simulink model "GCI_Ctrl_PLL_C2000"  (R2024a)
settings: Solver=FixedStepDiscrete  StartTime=0.0  StopTime=8  FixedStep=Sim.ContSampleTime  RelTol=1e-3  EnableMultiTasking=on
values from neighbouring files (symbols this model uses):
  ADPTV = 1.3912    [ModelDD.sldd]
  Ctrl = 0    [ModelDD.sldd]
  EnableMonitors = 0    [ModelDD.sldd]
  FrcPwr = 1    [ModelDD.sldd]
  IdSp = 0.0    [ModelDD.sldd]
  IqSp = 0.0    [ModelDD.sldd]
  ModReq = 1    [ModelDD.sldd]
  PorISel = 0    [ModelDD.sldd]
  PSp = 0.0    [ModelDD.sldd]
  QSp = 0.0    [ModelDD.sldd]
  Sim : value not decoded    [ModelDD.sldd]
  Test = 0    [ModelDD.sldd]
  Var = 650.0    [ModelDD.sldd]
undefined symbols (not defined in the file or in its folder): DiscIntNeverNeededParam, Down, GPTRIP1SEL, GPTRIP2SEL, magnitude, P, TZ1, TZ2, Up
libraries: simulink x38, c2837xDlib x22, c2802xlib x15, slpidlib x9, spsMeanLib x9, spsCurrentMeasurementLib x7, spsThreePhaseVIMeasurementLib x5, spsVoltageMeasurementLib x5, spsTHDLib x4, spsSeriesRLCBranchLib x4, svdutilitieslib x3, c280xlib x3
(part 4 of 11)

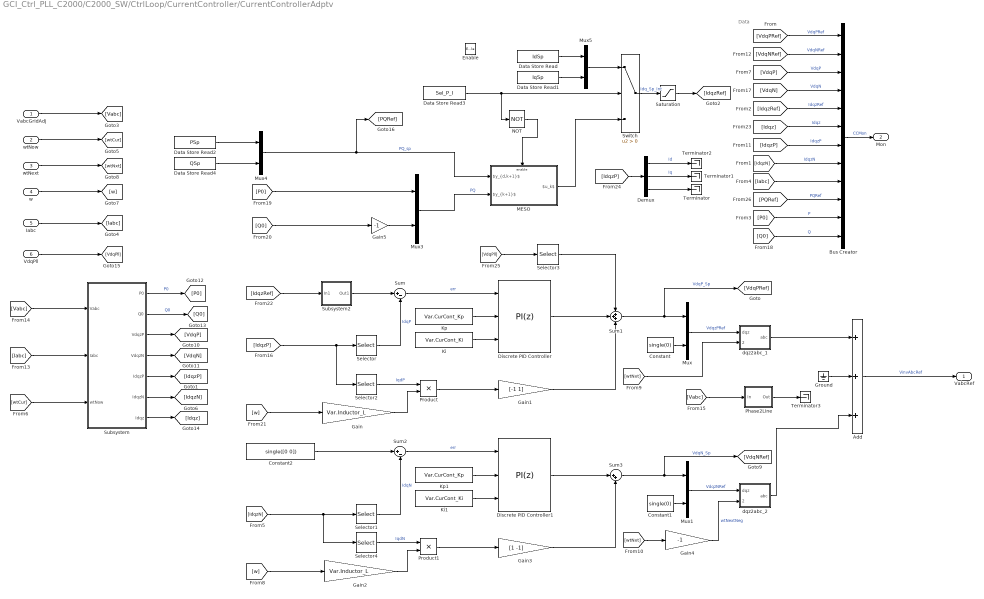
== system GCI_Ctrl_PLL_C2000/C2000_SW/CtrlLoop/CurrentController/CurrentControllerAdptv ==
  note: Data
  VabcGridAdj : Inport
  wtNow : Inport  Port=2
  wtNext : Inport  Port=3
  w : Inport  Port=4
  Iabc : Inport  Port=5
  VdqPll : Inport  Port=6
  Enable : EnablePort  StatesWhenEnabling=reset
  Add : Sum  Inputs=+++
  Bus Creator : BusCreator  Inputs=12
  Constant : Constant  Value=single(0)
  Constant1 : Constant  Value=single(0)
  Constant2 : Constant  Value=single([0 0])
  Data Store Read : DataStoreRead  DataStoreName=IdSp  IndexOptions=Index vector (dialog)  Indices=1  OutputSizes=1
  Data Store Read1 : DataStoreRead  DataStoreName=IqSp  IndexOptions=Index vector (dialog)  Indices=1  OutputSizes=1
  Data Store Read2 : DataStoreRead  DataStoreName=PSp  IndexOptions=Index vector (dialog)  Indices=1  OutputSizes=1
  Data Store Read3 : DataStoreRead  DataStoreName=Sel_P_I  IndexOptions=Index vector (dialog)  Indices=1  OutputSizes=1
  Data Store Read4 : DataStoreRead  DataStoreName=QSp  IndexOptions=Index vector (dialog)  Indices=1  OutputSizes=1
  Demux : Demux  Outputs=3
  Discrete PID Controller : slpidlib/PID Controller  Controller=PI  Form=Parallel  TimeDomain=Discrete-time  UseExternalTs=off  SampleTime=-1  IntegratorMethod=Forward Euler  FilterMethod=Forward Euler  ControllerParametersSource=external  P=1  I=1  UseKiTs=off  D=0  UseExternalDerivativeSource=off  N=100  UseFilter=on  TunerSelectOption=Transfer Function Based (PID Tuner App)  InitialConditionSource=internal  InitialConditionForIntegrator=0  InitialConditionForFilter=0  DifferentiatorICPrevScaledInput=0  ExternalReset=none  TrackingMode=off  Kt=1  LimitOutput=on  SatLimitsSource=internal  UpperSaturationLimit=Var.CurCont_MaxVdVq  LowerSaturationLimit=-Var.CurCont_MaxVdVq  LinearizeAsGain=on  AntiWindupMode=clamping  Kb=1  LimitIntegrator=off  UpperIntegratorSaturationLimit=inf  LowerIntegratorSaturationLimit=-inf  POutMin=[]  POutMax=[]  IOutMin=[]  IOutMax=[]  DOutMin=[]  DOutMax=[]  NOutMin=[]  NOutMax=[]  SumOutMin=[]  SumOutMax=[]  SaturationOutMin=[]  SaturationOutMax=[]  PParamMin=[]  PParamMax=[]  IParamMin=[]  IParamMax=[]  DParamMin=[]  DParamMax=[]  NParamMin=[]  NParamMax=[]  KbParamMin=[]  KbParamMax=[]  KtParamMin=[]  KtParamMax=[]  KbOutMin=[]  KbOutMax=[]  KtOutMin=[]  KtOutMax=[]  IntegratorOutMin=[]  IntegratorOutMax=[]  FilterOutMin=[]  FilterOutMax=[]  SumI1OutMin=[]  SumI1OutMax=[]  SumI2OutMin=[]  SumI2OutMax=[]  SumI3OutMin=[]  SumI3OutMax=[]  SumI4OutMin=[]  SumI4OutMax=[]  SumDOutMin=[]  SumDOutMax=[]  DifferentiatorOutMin=[]  DifferentiatorOutMax=[]  FilterDiffOutCoefMin=[]  FilterDiffOutCoefMax=[]  ReciprocalOutMin=[]  ReciprocalOutMax=[]  SumDenOutMin=[]  SumDenOutMax=[]  SumNumOutMin=[]  SumNumOutMax=[]  DivideOutMin=[]  DivideOutMax=[]  UdiffTsProdOutMin=[]  UdiffTsProdOutMax=[]  NTsProdOutMin=[]  NTsProdOutMax=[]  UintegralTsProdOutMin=[]  UintegralTsProdOutMax=[]  UngainTsProdOutMin=[]  UngainTsProdOutMax=[]  ClampingZeroOutDataTypeStr=Inherit: Inherit via back propagation  ClampingZeroOutMin=[]  ClampingZeroOutMax=[]  FilterDenConstantOutDataTypeStr=Inherit: Inherit via back propagation  FilterDenConstantOutMin=[]  FilterDenConstantOutMax=[]  PCopyOutDataTypeStr=Inherit: Inherit via back propagation  PCopyOutMin=[]  PCopyOutMax=[]  NCopyOutDataTypeStr=Inherit: Inherit via back propagation  NCopyOutMin=[]  NCopyOutMax=[]  IntegratorContinuousStateAttributes=''  IntegratorStateMustResolveToSignalObject=off  IntegratorRTWStateStorageClass=Auto  FilterContinuousStateAttributes=''  FilterStateMustResolveToSignalObject=off  FilterRTWStateStorageClass=Auto  ParallelPVariant=ExternalParameters  IdealPVariant=Disabled  IVariant=ExternalParameters  DVariant=Disabled  IntegratorVariant=Discrete  SatVariant=Enabled  AWVariant=DiscClampingParallel  PCopyVariant=Disabled  TRVariant=Disabled  FdbkBlocksVariant=Forward  IdealPFdbkVariant=Disabled  SatFdbkVariant=Disabled  DerivativeFilterVariant=Disabled  NVariant=Disabled  NCopyVariant=Disabled_SignalSpec  FilterICVariant=Disabled  IntegratorICVariant=InternalICs  ExternalResetVariant=Disabled  TRSumVariant=Passthrough  SumFdbkVariant=Disabled  SumVariant=Sum_PI  TsampFilterVariant=InternalTs  TsampNgainVariant=Passthrough  TsampIntegralVariant=Disabled_SignalSpec  ExternalSaturationOutDataTypeStr=Inherit: Same as second input  DerivativeSourceVariant=Disabled
  Discrete PID Controller1 : slpidlib/PID Controller  Controller=PI  Form=Parallel  TimeDomain=Discrete-time  UseExternalTs=off  SampleTime=-1  IntegratorMethod=Forward Euler  FilterMethod=Forward Euler  ControllerParametersSource=external  P=1  I=1  UseKiTs=off  D=0  UseExternalDerivativeSource=off  N=100  UseFilter=on  TunerSelectOption=Transfer Function Based (PID Tuner App)  InitialConditionSource=internal  InitialConditionForIntegrator=0  InitialConditionForFilter=0  DifferentiatorICPrevScaledInput=0  ExternalReset=none  TrackingMode=off  Kt=1  LimitOutput=on  SatLimitsSource=internal  UpperSaturationLimit=Var.CurCont_MaxVdVq  LowerSaturationLimit=-Var.CurCont_MaxVdVq  LinearizeAsGain=on  AntiWindupMode=clamping  Kb=1  LimitIntegrator=off  UpperIntegratorSaturationLimit=inf  LowerIntegratorSaturationLimit=-inf  POutMin=[]  POutMax=[]  IOutMin=[]  IOutMax=[]  DOutMin=[]  DOutMax=[]  NOutMin=[]  NOutMax=[]  SumOutMin=[]  SumOutMax=[]  SaturationOutMin=[]  SaturationOutMax=[]  PParamMin=[]  PParamMax=[]  IParamMin=[]  IParamMax=[]  DParamMin=[]  DParamMax=[]  NParamMin=[]  NParamMax=[]  KbParamMin=[]  KbParamMax=[]  KtParamMin=[]  KtParamMax=[]  KbOutMin=[]  KbOutMax=[]  KtOutMin=[]  KtOutMax=[]  IntegratorOutMin=[]  IntegratorOutMax=[]  FilterOutMin=[]  FilterOutMax=[]  SumI1OutMin=[]  SumI1OutMax=[]  SumI2OutMin=[]  SumI2OutMax=[]  SumI3OutMin=[]  SumI3OutMax=[]  SumI4OutMin=[]  SumI4OutMax=[]  SumDOutMin=[]  SumDOutMax=[]  DifferentiatorOutMin=[]  DifferentiatorOutMax=[]  FilterDiffOutCoefMin=[]  FilterDiffOutCoefMax=[]  ReciprocalOutMin=[]  ReciprocalOutMax=[]  SumDenOutMin=[]  SumDenOutMax=[]  SumNumOutMin=[]  SumNumOutMax=[]  DivideOutMin=[]  DivideOutMax=[]  UdiffTsProdOutMin=[]  UdiffTsProdOutMax=[]  NTsProdOutMin=[]  NTsProdOutMax=[]  UintegralTsProdOutMin=[]  UintegralTsProdOutMax=[]  UngainTsProdOutMin=[]  UngainTsProdOutMax=[]  ClampingZeroOutDataTypeStr=Inherit: Inherit via back propagation  ClampingZeroOutMin=[]  ClampingZeroOutMax=[]  FilterDenConstantOutDataTypeStr=Inherit: Inherit via back propagation  FilterDenConstantOutMin=[]  FilterDenConstantOutMax=[]  PCopyOutDataTypeStr=Inherit: Inherit via back propagation  PCopyOutMin=[]  PCopyOutMax=[]  NCopyOutDataTypeStr=Inherit: Inherit via back propagation  NCopyOutMin=[]  NCopyOutMax=[]  IntegratorContinuousStateAttributes=''  IntegratorStateMustResolveToSignalObject=off  IntegratorRTWStateStorageClass=Auto  FilterContinuousStateAttributes=''  FilterStateMustResolveToSignalObject=off  FilterRTWStateStorageClass=Auto  ParallelPVariant=ExternalParameters  IdealPVariant=Disabled  IVariant=ExternalParameters  DVariant=Disabled  IntegratorVariant=Discrete  SatVariant=Enabled  AWVariant=DiscClampingParallel  PCopyVariant=Disabled  TRVariant=Disabled  FdbkBlocksVariant=Forward  IdealPFdbkVariant=Disabled  SatFdbkVariant=Disabled  DerivativeFilterVariant=Disabled  NVariant=Disabled  NCopyVariant=Disabled_SignalSpec  FilterICVariant=Disabled  IntegratorICVariant=InternalICs  ExternalResetVariant=Disabled  TRSumVariant=Passthrough  SumFdbkVariant=Disabled  SumVariant=Sum_PI  TsampFilterVariant=InternalTs  TsampNgainVariant=Passthrough  TsampIntegralVariant=Disabled_SignalSpec  ExternalSaturationOutDataTypeStr=Inherit: Same as second input  DerivativeSourceVariant=Disabled
  Gain : Gain  Gain=Var.Inductor_L
  Gain1 : Gain  Gain=[-1 1]  ParamDataTypeStr=single
  Gain2 : Gain  Gain=Var.Inductor_L  ParamDataTypeStr=single
  Gain3 : Gain  Gain=[1 -1]  ParamDataTypeStr=single
  Gain4 : Gain  Gain=-1  ParamDataTypeStr=single
  Gain5 : Gain  Gain=-1  ParamDataTypeStr=single
  Ground : Ground
  Ki : Constant  Value=Var.CurCont_Ki
  Ki1 : Constant  Value=Var.CurCont_Ki
  Kp : Constant  Value=Var.CurCont_Kp
  Kp1 : Constant  Value=Var.CurCont_Kp
  MESO : Subsystem
  Mux{,1,3..5} (5 alike) : Mux  Inputs=2
  NOT : Logic  Operator=NOT  AllPortsSameDT=off  OutDataTypeStr=boolean
  Phase2Line : Subsystem  Variant=on  VariantControl=Subsystem2
  Product : Product
  Product1 : Product
  Saturation : Saturate  UpperLimit=100  LowerLimit=-100
  Selector : Selector  InputPortWidth=3  IndexOptions=Index vector (dialog)  Indices=[1 2]  OutputSizes=1
  Selector1 : Selector  InputPortWidth=3  IndexOptions=Index vector (dialog)  Indices=[1 2]  OutputSizes=1
  Selector2 : Selector  InputPortWidth=3  IndexOptions=Index vector (dialog)  Indices=[2 1]  OutputSizes=1
  Selector3 : Selector  InputPortWidth=3  IndexOptions=Index vector (dialog)  Indices=[1 2]  OutputSizes=1
  Selector4 : Selector  InputPortWidth=3  IndexOptions=Index vector (dialog)  Indices=[2 1]  OutputSizes=1
  Subsystem : Subsystem
  Subsystem2 : Subsystem
  Sum : Sum  Inputs=|+-
  Sum1 : Sum  Inputs=+++
  Sum2 : Sum  Inputs=|+-
  Sum3 : Sum  Inputs=|++
  Switch : Switch  Criteria=u2 > Threshold  SaturateOnIntegerOverflow=off  InputSameDT=off
  Terminator{,1..3} (4 alike) : Terminator
  dqz2abc_1 : Subsystem
  dqz2abc_2 : Subsystem
  VabcRef : Outport  VectorParamsAs1DForOutWhenUnconnected=off
  Mon : Outport  Port=2  VectorParamsAs1DForOutWhenUnconnected=off
  wires:
  Subsystem2/1(Out1) -> Sum/1
  [IdqzRef] -> Subsystem2/1(In1)
  Selector3/1 -> Sum1/1
  [wtCur] -> Subsystem/3(wtNow)
  [Vabc] -> Subsystem/1(Vabc)
  Ground/1 -> Add/2
  [VdqPll] -> Selector3/1
  VdqPll/1 -> [VdqPll]
  Data Store Read/1 -> Mux5/1
  Data Store Read1/1 -> Mux5/2
  Phase2Line/1(Out) -> Terminator3/1
  Demux/2 -> Terminator1/1  "Iq"
  Demux/1 -> Terminator2/1  "Id"
  Demux/3 -> Terminator/1
  [IdqzP] -> Demux/1
  wtNow/1 -> [wtCur]
  NOT/1 -> MESO/Enable
  MESO/1($u_k$) -> Switch/3
  Switch/1 -> Saturation/1  "Idq_Sp_Int"
  Data Store Read3/1 -> Switch/2, NOT/1
  Mux5/1 -> Switch/1
  [IdqzP] -> Bus Creator/7  "IdqzP"
  Subsystem/7(Idqz) -> [Idqz]
  Subsystem/6(IdqzN) -> [IdqzN]
  Subsystem/5(IdqzP) -> [IdqzP]
  Subsystem/3(VdqzP) -> [VdqP]
  Subsystem/4(VdqzN) -> [VdqN]
  [w] -> Gain/1
  [IdqzP] -> Selector2/1, Selector/1
  [Vabc] -> Phase2Line/1(In)
  [Iabc] -> Subsystem/2(Iabc)
  Subsystem/2(Q0) -> [Q0]  "Q0"
  Subsystem/1(P0) -> [P0]  "P0"
  Gain5/1 -> Mux3/2
  [Q0] -> Gain5/1
  [P0] -> Mux3/1
  Discrete PID Controller/1 -> Sum1/2
  [Q0] -> Bus Creator/12  "Q"
  [P0] -> Bus Creator/11  "P"
  [VdqN] -> Bus Creator/4  "VdqN"
  [VdqP] -> Bus Creator/3  "VdqP"
  [VdqNRef] -> Bus Creator/2  "VdqNRef"
  [IdqzN] -> Bus Creator/8  "IdqzN"
  [wtNxt] -> Gain4/1
  [wtNxt] -> dqz2abc_1/2(wtNext)
  [w] -> Gain2/1
  VabcGridAdj/1 -> [Vabc]
  Add/1 -> VabcRef/1  "VinvAbcRef"
  dqz2abc_2/1(abc) -> Add/3
  Gain4/1 -> dqz2abc_2/2(wtNext)  "wtNextNeg"
  w/1 -> [w]
  Ki1/1 -> Discrete PID Controller1/3
  Sum2/1 -> Discrete PID Controller1/1  "err"
  Constant2/1 -> Sum2/1
  Sum3/1 -> [VdqNRef], Mux1/1  "VdqN_Sp"
  Kp1/1 -> Discrete PID Controller1/2
  Selector4/1 -> Product1/1  "IqdN"
  Gain3/1 -> Sum3/2
  [IdqzN] -> Selector1/1, Selector4/1
  Product1/1 -> Gain3/1
  Gain2/1 -> Product1/2
  Selector1/1 -> Sum2/2  "IdqN"
  Constant1/1 -> Mux1/2
  Discrete PID Controller1/1 -> Sum3/1
  Mux1/1 -> dqz2abc_2/1(dqz)  "VdqzNRef"
  Sum/1 -> Discrete PID Controller/1  "err"
  Selector/1 -> Sum/2  "IdqP"
  Ki/1 -> Discrete PID Controller/3
  Sum1/1 -> [VdqPRef], Mux/1  "VdqP_Sp"
  Gain/1 -> Product/2
  Product/1 -> Gain1/1
  Selector2/1 -> Product/1  "IqdP"
  Gain1/1 -> Sum1/3
  Constant/1 -> Mux/2
  Iabc/1 -> [Iabc]
  wtNext/1 -> [wtNxt]
  Mux/1 -> dqz2abc_1/1(dqz)  "VdqzPRef"
  [Idqz] -> Bus Creator/6  "Idqz"
  [IdqzRef] -> Bus Creator/5  "IdqzRef"
  [VdqPRef] -> Bus Creator/1  "VdqPRef"
  Bus Creator/1 -> Mon/1  "CCMon"
  [Iabc] -> Bus Creator/9
  dqz2abc_1/1(abc) -> Add/1
  Mux3/1 -> MESO/2("$y_{k+1}$")  "PQ"
  Mux4/1 -> [PQRef], MESO/1("$y_{d,k+1}$")  "PQ_sp"
  Saturation/1 -> [IdqzRef]
  Data Store Read2/1 -> Mux4/1
  Data Store Read4/1 -> Mux4/2
  Kp/1 -> Discrete PID Controller/2
  [PQRef] -> Bus Creator/10  "PQRef"

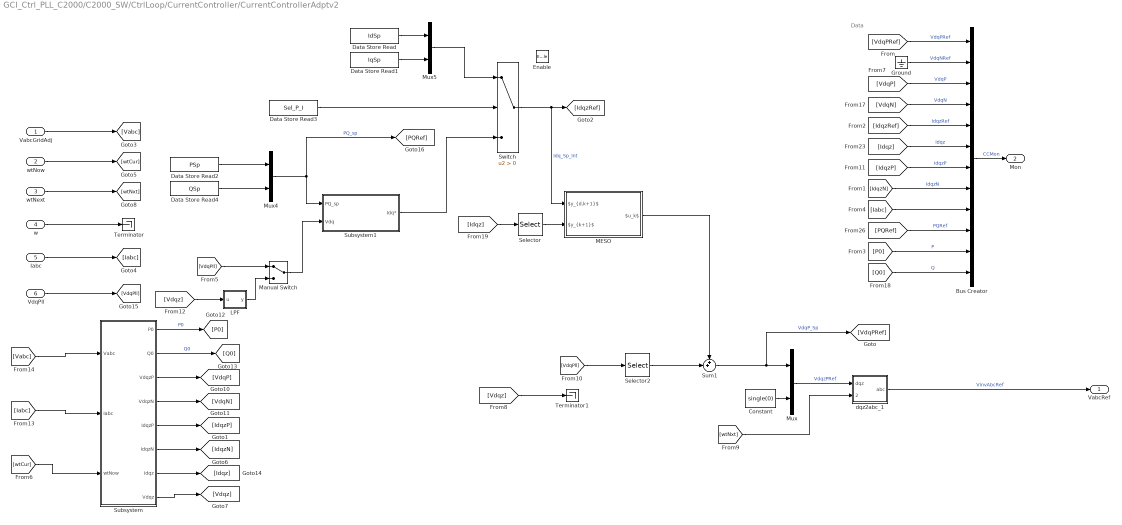
== system GCI_Ctrl_PLL_C2000/C2000_SW/CtrlLoop/CurrentController/CurrentControllerAdptv2 ==
  note: Data
  VabcGridAdj : Inport
  wtNow : Inport  Port=2
  wtNext : Inport  Port=3
  w : Inport  Port=4
  Iabc : Inport  Port=5
  VdqPll : Inport  Port=6
  Enable : EnablePort  StatesWhenEnabling=reset
  Bus Creator : BusCreator  Inputs=12
  Constant : Constant  Value=single(0)
  Data Store Read : DataStoreRead  DataStoreName=IdSp  IndexOptions=Index vector (dialog)  Indices=1  OutputSizes=1
  Data Store Read1 : DataStoreRead  DataStoreName=IqSp  IndexOptions=Index vector (dialog)  Indices=1  OutputSizes=1
  Data Store Read2 : DataStoreRead  DataStoreName=PSp  IndexOptions=Index vector (dialog)  Indices=1  OutputSizes=1
  Data Store Read3 : DataStoreRead  DataStoreName=Sel_P_I  IndexOptions=Index vector (dialog)  Indices=1  OutputSizes=1
  Data Store Read4 : DataStoreRead  DataStoreName=QSp  IndexOptions=Index vector (dialog)  Indices=1  OutputSizes=1
  Ground : Ground
  LPF : Subsystem  mask{Ts=1/(Var.PWM_Freq), w=single(2*pi*20), K=single(1), y_0=0}
      mask prompts: Ts "Sample Time (s)"; w "CutOff Freq (-3db) (rad/s)"; K "Gain"; y_0 "Initial output"
  MESO : Subsystem
  Manual Switch : ManualSwitch
  Mux : Mux  Inputs=2
  Mux4 : Mux  Inputs=2
  Mux5 : Mux  Inputs=2
  Selector : Selector  InputPortWidth=3  IndexOptions=Index vector (dialog)  Indices=[1 2]  OutputSizes=1
  Selector2 : Selector  InputPortWidth=3  IndexOptions=Index vector (dialog)  Indices=[1 2]  OutputSizes=1
  Subsystem : Subsystem
  Subsystem1 : Subsystem
  Sum1 : Sum  Inputs=++|
  Switch : Switch  Criteria=u2 > Threshold  SaturateOnIntegerOverflow=off  InputSameDT=off
  Terminator : Terminator
  Terminator1 : Terminator
  dqz2abc_1 : Subsystem
  VabcRef : Outport  VectorParamsAs1DForOutWhenUnconnected=off
  Mon : Outport  Port=2  VectorParamsAs1DForOutWhenUnconnected=off
  wires:
  [PQRef] -> Bus Creator/10  "PQRef"
  Data Store Read4/1 -> Mux4/2
  Data Store Read2/1 -> Mux4/1
  Mux4/1 -> Subsystem1/1(PQ_sp), [PQRef]  "PQ_sp"
  [Iabc] -> Bus Creator/9
  Bus Creator/1 -> Mon/1  "CCMon"
  [VdqPRef] -> Bus Creator/1  "VdqPRef"
  [IdqzRef] -> Bus Creator/5  "IdqzRef"
  [Idqz] -> Bus Creator/6  "Idqz"
  Mux/1 -> dqz2abc_1/1(dqz)  "VdqzPRef"
  wtNext/1 -> [wtNxt]
  Iabc/1 -> [Iabc]
  Constant/1 -> Mux/2
  Sum1/1 -> Mux/1, [VdqPRef]  "VdqP_Sp"
  w/1 -> Terminator/1
  dqz2abc_1/1(abc) -> VabcRef/1  "VinvAbcRef"
  VabcGridAdj/1 -> [Vabc]
  [wtNxt] -> dqz2abc_1/2(wtNext)
  [IdqzN] -> Bus Creator/8  "IdqzN"
  Ground/1 -> Bus Creator/2  "VdqNRef"
  [VdqP] -> Bus Creator/3  "VdqP"
  [VdqN] -> Bus Creator/4  "VdqN"
  [P0] -> Bus Creator/11  "P"
  [Q0] -> Bus Creator/12  "Q"
  Subsystem/1(P0) -> [P0]  "P0"
  Subsystem/2(Q0) -> [Q0]  "Q0"
  [Iabc] -> Subsystem/2(Iabc)
  Subsystem/4(VdqzN) -> [VdqN]
  Subsystem/3(VdqzP) -> [VdqP]
  Subsystem/5(IdqzP) -> [IdqzP]
  Subsystem/6(IdqzN) -> [IdqzN]
  Subsystem/7(Idqz) -> [Idqz]
  [IdqzP] -> Bus Creator/7  "IdqzP"
  Mux5/1 -> Switch/1
  Data Store Read3/1 -> Switch/2
  Switch/1 -> [IdqzRef], MESO/1("$y_{d,k+1}$")  "Idq_Sp_Int"
  wtNow/1 -> [wtCur]
  Data Store Read1/1 -> Mux5/2
  Data Store Read/1 -> Mux5/1
  VdqPll/1 -> [VdqPll]
  [Vabc] -> Subsystem/1(Vabc)
  [wtCur] -> Subsystem/3(wtNow)
  [Idqz] -> Selector/1
  Selector/1 -> MESO/2("$y_{k+1}$")
  [VdqPll] -> Selector2/1
  Selector2/1 -> Sum1/2
  MESO/1($u_k$) -> Sum1/1
  Subsystem/8(Vdqz) -> [Vdqz]
  Manual Switch/1 -> Subsystem1/2(Vdq)
  Subsystem1/1(Idq*) -> Switch/3
  [Vdqz] -> Terminator1/1
  [VdqPll] -> Manual Switch/1
  [Vdqz] -> LPF/1(u)
  LPF/1(y) -> Manual Switch/2

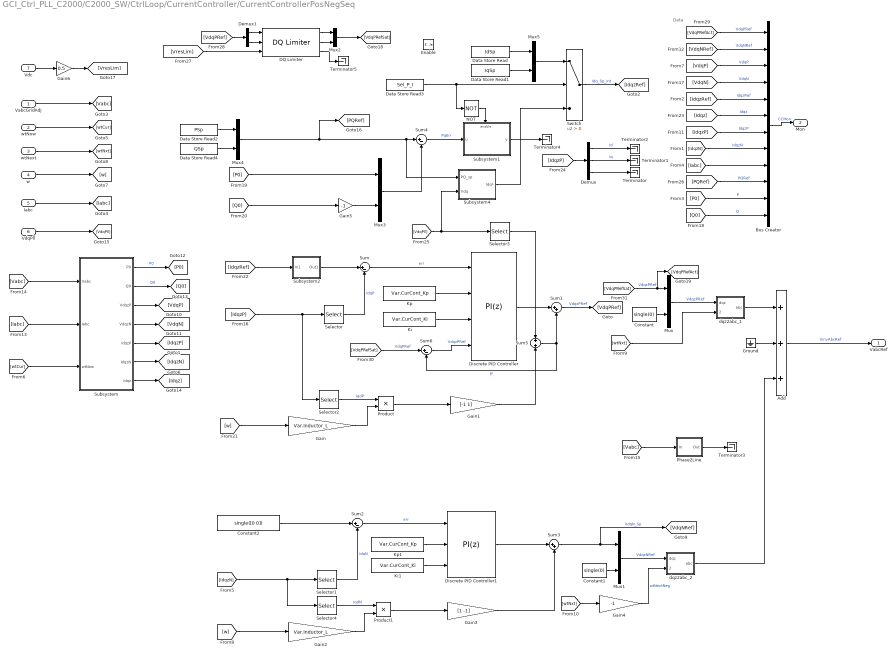
== system GCI_Ctrl_PLL_C2000/C2000_SW/CtrlLoop/CurrentController/CurrentControllerPosNegSeq ==
  note: Data
  VabcGridAdj : Inport
  wtNow : Inport  Port=2
  wtNext : Inport  Port=3
  w : Inport  Port=4
  Iabc : Inport  Port=5
  VdqPll : Inport  Port=6
  Vdc : Inport  Port=7
  Enable : EnablePort  StatesWhenEnabling=reset
  Add : Sum  Inputs=+++
  Bus Creator : BusCreator  Inputs=12
  Constant : Constant  Value=single(0)
  Constant1 : Constant  Value=single(0)
  Constant2 : Constant  Value=single([0 0])
  DQ Limiter : mcbcontrolslib/DQ Limiter  satMethodInputType=Specify via dialog  satMethodSelected=D-Q equivalence  satLimitInputType=Input port  Vmax=1
      settings: LibrarySourceBlock=mcbhdllib/Controls/Control Reference/DQ Limiter
  Data Store Read : DataStoreRead  DataStoreName=IdSp  IndexOptions=Index vector (dialog)  Indices=1  OutputSizes=1
  Data Store Read1 : DataStoreRead  DataStoreName=IqSp  IndexOptions=Index vector (dialog)  Indices=1  OutputSizes=1
  Data Store Read2 : DataStoreRead  DataStoreName=PSp  IndexOptions=Index vector (dialog)  Indices=1  OutputSizes=1
  Data Store Read3 : DataStoreRead  DataStoreName=Sel_P_I  IndexOptions=Index vector (dialog)  Indices=1  OutputSizes=1
  Data Store Read4 : DataStoreRead  DataStoreName=QSp  IndexOptions=Index vector (dialog)  Indices=1  OutputSizes=1
  Demux : Demux  Outputs=3
  Demux1 : Demux  Outputs=2
  Discrete PID Controller : slpidlib/PID Controller  Controller=PI  Form=Parallel  TimeDomain=Discrete-time  UseExternalTs=off  SampleTime=-1  IntegratorMethod=Forward Euler  FilterMethod=Forward Euler  ControllerParametersSource=external  P=1  I=1  UseKiTs=off  D=0  UseExternalDerivativeSource=off  N=100  UseFilter=on  TunerSelectOption=Transfer Function Based (PID Tuner App)  InitialConditionSource=internal  InitialConditionForIntegrator=0  InitialConditionForFilter=0  DifferentiatorICPrevScaledInput=0  ExternalReset=none  TrackingMode=on  Kt=single(1/Var.PWM_Freq)  LimitOutput=off  SatLimitsSource=external  UpperSaturationLimit=Var.CurCont_MaxVdVq  LowerSaturationLimit=-Var.CurCont_MaxVdVq  LinearizeAsGain=on  AntiWindupMode=clamping  Kb=1  LimitIntegrator=off  UpperIntegratorSaturationLimit=inf  LowerIntegratorSaturationLimit=-inf  POutMin=[]  POutMax=[]  IOutMin=[]  IOutMax=[]  DOutMin=[]  DOutMax=[]  NOutMin=[]  NOutMax=[]  SumOutMin=[]  SumOutMax=[]  SaturationOutMin=[]  SaturationOutMax=[]  PParamMin=[]  PParamMax=[]  IParamMin=[]  IParamMax=[]  DParamMin=[]  DParamMax=[]  NParamMin=[]  NParamMax=[]  KbParamMin=[]  KbParamMax=[]  KtParamMin=[]  KtParamMax=[]  KbOutMin=[]  KbOutMax=[]  KtOutMin=[]  KtOutMax=[]  IntegratorOutMin=[]  IntegratorOutMax=[]  FilterOutMin=[]  FilterOutMax=[]  SumI1OutMin=[]  SumI1OutMax=[]  SumI2OutMin=[]  SumI2OutMax=[]  SumI3OutMin=[]  SumI3OutMax=[]  SumI4OutMin=[]  SumI4OutMax=[]  SumDOutMin=[]  SumDOutMax=[]  DifferentiatorOutMin=[]  DifferentiatorOutMax=[]  FilterDiffOutCoefMin=[]  FilterDiffOutCoefMax=[]  ReciprocalOutMin=[]  ReciprocalOutMax=[]  SumDenOutMin=[]  SumDenOutMax=[]  SumNumOutMin=[]  SumNumOutMax=[]  DivideOutMin=[]  DivideOutMax=[]  UdiffTsProdOutMin=[]  UdiffTsProdOutMax=[]  NTsProdOutMin=[]  NTsProdOutMax=[]  UintegralTsProdOutMin=[]  UintegralTsProdOutMax=[]  UngainTsProdOutMin=[]  UngainTsProdOutMax=[]  ClampingZeroOutDataTypeStr=Inherit: Inherit via back propagation  ClampingZeroOutMin=[]  ClampingZeroOutMax=[]  FilterDenConstantOutDataTypeStr=Inherit: Inherit via back propagation  FilterDenConstantOutMin=[]  FilterDenConstantOutMax=[]  PCopyOutDataTypeStr=Inherit: Inherit via back propagation  PCopyOutMin=[]  PCopyOutMax=[]  NCopyOutDataTypeStr=Inherit: Inherit via back propagation  NCopyOutMin=[]  NCopyOutMax=[]  IntegratorContinuousStateAttributes=''  IntegratorStateMustResolveToSignalObject=off  IntegratorRTWStateStorageClass=Auto  FilterContinuousStateAttributes=''  FilterStateMustResolveToSignalObject=off  FilterRTWStateStorageClass=Auto  ParallelPVariant=ExternalParameters  IdealPVariant=Disabled  IVariant=ExternalParameters  DVariant=Disabled  IntegratorVariant=Discrete  SatVariant=Disabled  AWVariant=Passthrough  PCopyVariant=Disabled  TRVariant=Enabled  FdbkBlocksVariant=Forward  IdealPFdbkVariant=Disabled  SatFdbkVariant=Disabled  DerivativeFilterVariant=Disabled  NVariant=Disabled  NCopyVariant=Disabled_SignalSpec  FilterICVariant=Disabled  IntegratorICVariant=InternalICs  ExternalResetVariant=Disabled  TRSumVariant=TrackingMode  SumFdbkVariant=Disabled  SumVariant=Sum_PI  TsampFilterVariant=InternalTs  TsampNgainVariant=Passthrough  TsampIntegralVariant=Disabled_SignalSpec  ExternalSaturationOutDataTypeStr=Inherit: Same as second input  DerivativeSourceVariant=Disabled
  Discrete PID Controller1 : slpidlib/PID Controller  Controller=PI  Form=Parallel  TimeDomain=Discrete-time  UseExternalTs=off  SampleTime=-1  IntegratorMethod=Forward Euler  FilterMethod=Forward Euler  ControllerParametersSource=external  P=1  I=1  UseKiTs=off  D=0  UseExternalDerivativeSource=off  N=100  UseFilter=on  TunerSelectOption=Transfer Function Based (PID Tuner App)  InitialConditionSource=internal  InitialConditionForIntegrator=0  InitialConditionForFilter=0  DifferentiatorICPrevScaledInput=0  ExternalReset=none  TrackingMode=off  Kt=1  LimitOutput=on  SatLimitsSource=internal  UpperSaturationLimit=Var.CurCont_MaxVdVq  LowerSaturationLimit=-Var.CurCont_MaxVdVq  LinearizeAsGain=on  AntiWindupMode=clamping  Kb=1  LimitIntegrator=off  UpperIntegratorSaturationLimit=inf  LowerIntegratorSaturationLimit=-inf  POutMin=[]  POutMax=[]  IOutMin=[]  IOutMax=[]  DOutMin=[]  DOutMax=[]  NOutMin=[]  NOutMax=[]  SumOutMin=[]  SumOutMax=[]  SaturationOutMin=[]  SaturationOutMax=[]  PParamMin=[]  PParamMax=[]  IParamMin=[]  IParamMax=[]  DParamMin=[]  DParamMax=[]  NParamMin=[]  NParamMax=[]  KbParamMin=[]  KbParamMax=[]  KtParamMin=[]  KtParamMax=[]  KbOutMin=[]  KbOutMax=[]  KtOutMin=[]  KtOutMax=[]  IntegratorOutMin=[]  IntegratorOutMax=[]  FilterOutMin=[]  FilterOutMax=[]  SumI1OutMin=[]  SumI1OutMax=[]  SumI2OutMin=[]  SumI2OutMax=[]  SumI3OutMin=[]  SumI3OutMax=[]  SumI4OutMin=[]  SumI4OutMax=[]  SumDOutMin=[]  SumDOutMax=[]  DifferentiatorOutMin=[]  DifferentiatorOutMax=[]  FilterDiffOutCoefMin=[]  FilterDiffOutCoefMax=[]  ReciprocalOutMin=[]  ReciprocalOutMax=[]  SumDenOutMin=[]  SumDenOutMax=[]  SumNumOutMin=[]  SumNumOutMax=[]  DivideOutMin=[]  DivideOutMax=[]  UdiffTsProdOutMin=[]  UdiffTsProdOutMax=[]  NTsProdOutMin=[]  NTsProdOutMax=[]  UintegralTsProdOutMin=[]  UintegralTsProdOutMax=[]  UngainTsProdOutMin=[]  UngainTsProdOutMax=[]  ClampingZeroOutDataTypeStr=Inherit: Inherit via back propagation  ClampingZeroOutMin=[]  ClampingZeroOutMax=[]  FilterDenConstantOutDataTypeStr=Inherit: Inherit via back propagation  FilterDenConstantOutMin=[]  FilterDenConstantOutMax=[]  PCopyOutDataTypeStr=Inherit: Inherit via back propagation  PCopyOutMin=[]  PCopyOutMax=[]  NCopyOutDataTypeStr=Inherit: Inherit via back propagation  NCopyOutMin=[]  NCopyOutMax=[]  IntegratorContinuousStateAttributes=''  IntegratorStateMustResolveToSignalObject=off  IntegratorRTWStateStorageClass=Auto  FilterContinuousStateAttributes=''  FilterStateMustResolveToSignalObject=off  FilterRTWStateStorageClass=Auto  ParallelPVariant=ExternalParameters  IdealPVariant=Disabled  IVariant=ExternalParameters  DVariant=Disabled  IntegratorVariant=Discrete  SatVariant=Enabled  AWVariant=DiscClampingParallel  PCopyVariant=Disabled  TRVariant=Disabled  FdbkBlocksVariant=Forward  IdealPFdbkVariant=Disabled  SatFdbkVariant=Disabled  DerivativeFilterVariant=Disabled  NVariant=Disabled  NCopyVariant=Disabled_SignalSpec  FilterICVariant=Disabled  IntegratorICVariant=InternalICs  ExternalResetVariant=Disabled  TRSumVariant=Passthrough  SumFdbkVariant=Disabled  SumVariant=Sum_PI  TsampFilterVariant=InternalTs  TsampNgainVariant=Passthrough  TsampIntegralVariant=Disabled_SignalSpec  ExternalSaturationOutDataTypeStr=Inherit: Same as second input  DerivativeSourceVariant=Disabled
  Gain : Gain  Gain=Var.Inductor_L
  Gain1 : Gain  Gain=[-1 1]  ParamDataTypeStr=single
  Gain2 : Gain  Gain=Var.Inductor_L  ParamDataTypeStr=single
  Gain3 : Gain  Gain=[1 -1]  ParamDataTypeStr=single
  Gain4 : Gain  Gain=-1  ParamDataTypeStr=single
  Gain5 : Gain  Gain=-1  ParamDataTypeStr=single
  Gain6 : Gain  Gain=0.5
  Ground : Ground
  Ki : Constant  Value=Var.CurCont_Ki
  Ki1 : Constant  Value=Var.CurCont_Ki
  Kp : Constant  Value=Var.CurCont_Kp
  Kp1 : Constant  Value=Var.CurCont_Kp
  Mux{,1..5} (6 alike) : Mux  Inputs=2
  NOT : Logic  Operator=NOT  AllPortsSameDT=off  OutDataTypeStr=boolean
  Phase2Line : Subsystem  Variant=on  VariantControl=Subsystem2
  Product : Product
  Product1 : Product
  Selector : Selector  InputPortWidth=3  IndexOptions=Index vector (dialog)  Indices=[1 2]  OutputSizes=1
  Selector1 : Selector  InputPortWidth=3  IndexOptions=Index vector (dialog)  Indices=[1 2]  OutputSizes=1
  Selector2 : Selector  InputPortWidth=3  IndexOptions=Index vector (dialog)  Indices=[2 1]  OutputSizes=1
  Selector3 : Selector  InputPortWidth=3  IndexOptions=Index vector (dialog)  Indices=[1 2]  OutputSizes=1
  Selector4 : Selector  InputPortWidth=3  IndexOptions=Index vector (dialog)  Indices=[2 1]  OutputSizes=1
  Subsystem : Subsystem
  Subsystem1 : Subsystem
  Subsystem2 : Subsystem
  Subsystem4 : Subsystem
  Sum{,2,4,6} (4 alike) : Sum  Inputs=|+-
  Sum1 : Sum  Inputs=|++
  Sum3 : Sum  Inputs=|++
  Sum5 : Sum  Inputs=+||+
  Switch : Switch  Criteria=u2 > Threshold  SaturateOnIntegerOverflow=off  InputSameDT=off
  Terminator{,1..5} (6 alike) : Terminator
  dqz2abc_1 : Subsystem
  dqz2abc_2 : Subsystem
  VabcRef : Outport  VectorParamsAs1DForOutWhenUnconnected=off
  Mon : Outport  Port=2  VectorParamsAs1DForOutWhenUnconnected=off
  wires:
  dqz2abc_1/1(abc) -> Add/1
  [Iabc] -> Bus Creator/9
  Bus Creator/1 -> Mon/1  "CCMon"
  [VdqPRefAct] -> Bus Creator/1  "VdqPRef"
  [IdqzRef] -> Bus Creator/5  "IdqzRef"
  [Idqz] -> Bus Creator/6  "Idqz"
  Mux/1 -> dqz2abc_1/1(dqz)  "VdqzPRef"
  wtNext/1 -> [wtNxt]
  Iabc/1 -> [Iabc]
  Constant/1 -> Mux/2
  Gain1/1 -> Sum5/2
  Selector2/1 -> Product/1  "IqdP"
  Product/1 -> Gain1/1
  Gain/1 -> Product/2
  [VdqPRefSat] -> [VdqPRefAct], Mux/1  "VdqzPRef"
  Ki/1 -> Discrete PID Controller/3
  Selector/1 -> Sum/2  "IdqP"
  Kp/1 -> Discrete PID Controller/2
  Sum/1 -> Discrete PID Controller/1  "err"
  Mux1/1 -> dqz2abc_2/1(dqz)  "VdqzNRef"
  Discrete PID Controller1/1 -> Sum3/1
  Constant1/1 -> Mux1/2
  Selector1/1 -> Sum2/2  "IdqN"
  Gain2/1 -> Product1/2
  Product1/1 -> Gain3/1
  [IdqzN] -> Selector4/1, Selector1/1
  Gain3/1 -> Sum3/2
  Selector4/1 -> Product1/1  "IqdN"
  Kp1/1 -> Discrete PID Controller1/2
  Sum3/1 -> [VdqNRef], Mux1/1  "VdqN_Sp"
  Constant2/1 -> Sum2/1
  Sum2/1 -> Discrete PID Controller1/1  "err"
  Ki1/1 -> Discrete PID Controller1/3
  w/1 -> [w]
  Gain4/1 -> dqz2abc_2/2(wtNext)  "wtNextNeg"
  dqz2abc_2/1(abc) -> Add/3
  Add/1 -> VabcRef/1  "VinvAbcRef"
  VabcGridAdj/1 -> [Vabc]
  [w] -> Gain2/1
  [wtNxt] -> dqz2abc_1/2(wtNext)
  [wtNxt] -> Gain4/1
  [IdqzN] -> Bus Creator/8  "IdqzN"
  [VdqNRef] -> Bus Creator/2  "VdqNRef"
  [VdqP] -> Bus Creator/3  "VdqP"
  [VdqN] -> Bus Creator/4  "VdqN"
  [P0] -> Bus Creator/11  "P"
  [Q0] -> Bus Creator/12  "Q"
  Discrete PID Controller/1 -> Sum1/1
  [P0] -> Mux3/1
  [Q0] -> Gain5/1
  Mux3/1 -> Sum4/2
  Mux4/1 -> [PQRef], Subsystem4/1(PQ_sp), Sum4/1
  Gain5/1 -> Mux3/2
  Subsystem/1(P0) -> [P0]  "P0"
  Subsystem/2(Q0) -> [Q0]  "Q0"
  [Iabc] -> Subsystem/2(Iabc)
  [Vabc] -> Phase2Line/1(In)
  [IdqzP] -> Selector/1, Selector2/1
  [w] -> Gain/1
  Subsystem/4(VdqzN) -> [VdqN]
  Subsystem/3(VdqzP) -> [VdqP]
  Subsystem/5(IdqzP) -> [IdqzP]
  Subsystem/6(IdqzN) -> [IdqzN]
  Subsystem/7(Idqz) -> [Idqz]
  [IdqzP] -> Bus Creator/7  "IdqzP"
  Mux5/1 -> Switch/1
  Data Store Read3/1 -> NOT/1, Switch/2
  Switch/1 -> [IdqzRef]  "Idq_Sp_Int"
  Sum4/1 -> Subsystem1/1(u)  "PqErr"
  Subsystem4/1(Idq*) -> Switch/3
  NOT/1 -> Subsystem1/Enable
  wtNow/1 -> [wtCur]
  [IdqzP] -> Demux/1
  Demux/3 -> Terminator/1
  Demux/1 -> Terminator2/1  "Id"
  Demux/2 -> Terminator1/1  "Iq"
  Phase2Line/1(Out) -> Terminator3/1
  Data Store Read2/1 -> Mux4/1
  Data Store Read4/1 -> Mux4/2
  Data Store Read1/1 -> Mux5/2
  Data Store Read/1 -> Mux5/1
  VdqPll/1 -> [VdqPll]
  [VdqPll] -> Subsystem4/2(Vdq), Selector3/1
  Ground/1 -> Add/2
  [Vabc] -> Subsystem/1(Vabc)
  [wtCur] -> Subsystem/3(wtNow)
  Selector3/1 -> Sum5/1
  [IdqzRef] -> Subsystem2/1(In1)
  Subsystem2/1(Out1) -> Sum/1
  [PQRef] -> Bus Creator/10  "PQRef"
  Subsystem1/1(y) -> Terminator4/1
  Vdc/1 -> Gain6/1
  Gain6/1 -> [VresLim]
  [VresLim] -> DQ Limiter/3
  Demux1/2 -> DQ Limiter/2
  Demux1/1 -> DQ Limiter/1
  [VdqPRef] -> Demux1/1
  DQ Limiter/1 -> Mux2/1
  DQ Limiter/2 -> Mux2/2
  Mux2/1 -> [VdqPRefSat]
  Sum5/1 -> Sum6/2, Sum1/2  "ff"
  [VdqPRefSat] -> Sum6/1  "VdqPRef"
  Sum6/1 -> Discrete PID Controller/4  "VdqzPRef"
  Sum1/1 -> [VdqPRef]  "VdqzPRef"
  DQ Limiter/3 -> Terminator5/1

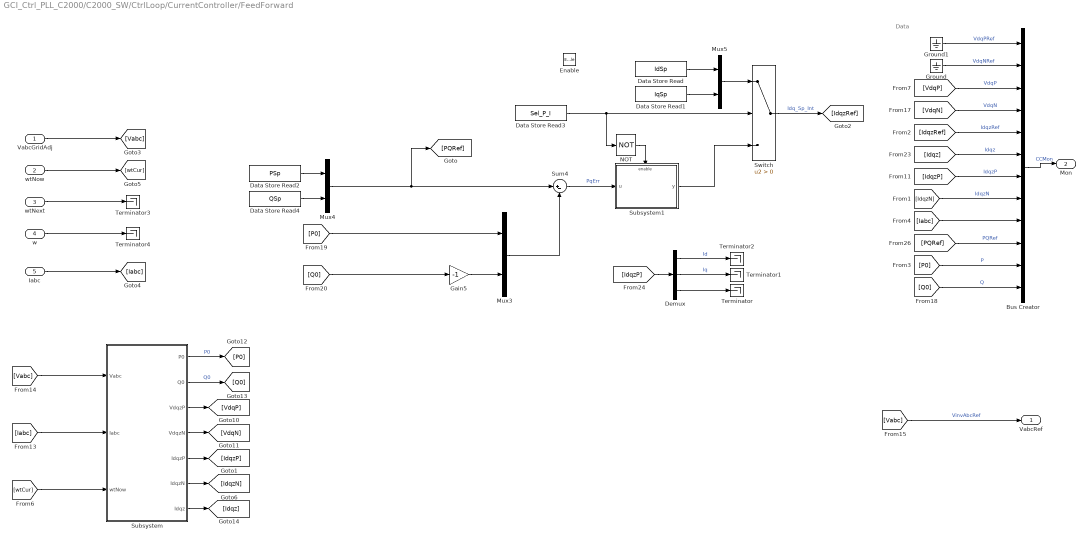
== system GCI_Ctrl_PLL_C2000/C2000_SW/CtrlLoop/CurrentController/FeedForward ==
  note: Data
  VabcGridAdj : Inport
  wtNow : Inport  Port=2
  wtNext : Inport  Port=3
  w : Inport  Port=4
  Iabc : Inport  Port=5
  Enable : EnablePort  StatesWhenEnabling=reset
  Bus Creator : BusCreator  Inputs=12
  Data Store Read : DataStoreRead  DataStoreName=IdSp  IndexOptions=Index vector (dialog)  Indices=1  OutputSizes=1
  Data Store Read1 : DataStoreRead  DataStoreName=IqSp  IndexOptions=Index vector (dialog)  Indices=1  OutputSizes=1
  Data Store Read2 : DataStoreRead  DataStoreName=PSp  IndexOptions=Index vector (dialog)  Indices=1  OutputSizes=1
  Data Store Read3 : DataStoreRead  DataStoreName=Sel_P_I  IndexOptions=Index vector (dialog)  Indices=1  OutputSizes=1
  Data Store Read4 : DataStoreRead  DataStoreName=QSp  IndexOptions=Index vector (dialog)  Indices=1  OutputSizes=1
  Demux : Demux  Outputs=3
  Gain5 : Gain  Gain=-1  ParamDataTypeStr=single
  Ground : Ground
  Ground1 : Ground
  Mux3 : Mux  Inputs=2
  Mux4 : Mux  Inputs=2
  Mux5 : Mux  Inputs=2
  NOT : Logic  Operator=NOT  AllPortsSameDT=off  OutDataTypeStr=boolean
  Subsystem : Subsystem
  Subsystem1 : Subsystem
  Sum4 : Sum  Inputs=|+-
  Switch : Switch  Criteria=u2 > Threshold  SaturateOnIntegerOverflow=off  InputSameDT=off
  Terminator{,1..4} (5 alike) : Terminator
  VabcRef : Outport  VectorParamsAs1DForOutWhenUnconnected=off
  Mon : Outport  Port=2  VectorParamsAs1DForOutWhenUnconnected=off
  wires:
  Ground/1 -> Bus Creator/2  "VdqNRef"
  [IdqzN] -> Bus Creator/8  "IdqzN"
  Switch/1 -> [IdqzRef]  "Idq_Sp_Int"
  [IdqzP] -> Bus Creator/7  "IdqzP"
  [P0] -> Bus Creator/11  "P"
  Subsystem1/1(y) -> Switch/3
  [wtCur] -> Subsystem/3(wtNow)
  Sum4/1 -> Subsystem1/1(u)  "PqErr"
  [Idqz] -> Bus Creator/6  "Idqz"
  [VdqN] -> Bus Creator/4  "VdqN"
  Subsystem/7(Idqz) -> [Idqz]
  Data Store Read3/1 -> NOT/1, Switch/2
  Gain5/1 -> Mux3/2
  [Iabc] -> Subsystem/2(Iabc)
  NOT/1 -> Subsystem1/Enable
  [IdqzP] -> Demux/1
  [Iabc] -> Bus Creator/9
  Subsystem/4(VdqzN) -> [VdqN]
  Subsystem/5(IdqzP) -> [IdqzP]
  [VdqP] -> Bus Creator/3  "VdqP"
  Bus Creator/1 -> Mon/1  "CCMon"
  Demux/2 -> Terminator1/1  "Iq"
  Subsystem/2(Q0) -> [Q0]  "Q0"
  w/1 -> Terminator4/1
  Iabc/1 -> [Iabc]
  Ground1/1 -> Bus Creator/1  "VdqPRef"
  [IdqzRef] -> Bus Creator/5  "IdqzRef"
  wtNow/1 -> [wtCur]
  Mux3/1 -> Sum4/2
  Subsystem/1(P0) -> [P0]  "P0"
  Subsystem/3(VdqzP) -> [VdqP]
  [P0] -> Mux3/1
  Subsystem/6(IdqzN) -> [IdqzN]
  wtNext/1 -> Terminator3/1
  [Q0] -> Gain5/1
  Demux/3 -> Terminator/1
  [Vabc] -> VabcRef/1  "VinvAbcRef"
  Mux5/1 -> Switch/1
  Demux/1 -> Terminator2/1  "Id"
  VabcGridAdj/1 -> [Vabc]
  [Q0] -> Bus Creator/12  "Q"
  [Vabc] -> Subsystem/1(Vabc)
  Data Store Read4/1 -> Mux4/2
  Data Store Read2/1 -> Mux4/1
  Mux4/1 -> [PQRef], Sum4/1
  Data Store Read/1 -> Mux5/1
  Data Store Read1/1 -> Mux5/2
  [PQRef] -> Bus Creator/10  "PQRef"

== system GCI_Ctrl_PLL_C2000/C2000_SW/CtrlLoop/Modulation/M_Adaptive ==
  note: Data Collection
  Vdc : Inport
  VabcSp : Inport  Port=2
  Enable : EnablePort  StatesWhenEnabling=reset
  Add : Sum
  Bus Creator : BusCreator  Inputs=4
  Constant : Constant  Value=50  OutDataTypeStr=single
  Discrete Transfer Fcn1 : DiscreteTransferFcn  Numerator=Var.Filt.Sec.num  Denominator=Var.Filt.Sec.den
  Divide : Product  Inputs=*/
  Gain : Gain  Gain=2  ParamDataTypeStr=single
  Gain1 : Gain  Gain=0.5  ParamDataTypeStr=single
  Gain2 : Gain  Gain=single(1/2)  ParamDataTypeStr=single
  Gain3 : Gain  Gain=50  ParamDataTypeStr=single  OutDataTypeStr=single
  Max : MinMax  Function=max
  Min : MinMax
  Product : Product
  Product1 : Product
  Relay : Relay  OnSwitchValue=single(0.8/sqrt(2))  OffSwitchValue=single(0.6/sqrt(2))
  Saturation : Saturate  UpperLimit=single(1000)  LowerLimit=single(1)
  Saturation1 : Saturate  UpperLimit=100  LowerLimit=0  OutDataTypeStr=single
  Sqrt : Sqrt
  Square : Math  Operator=square  SignedPower=on
  Sum : Sum  Inputs=|+-
  Sum1 : Sum  Inputs=|++  OutDataTypeStr=single
  Duty : Outport  VectorParamsAs1DForOutWhenUnconnected=off
  Mon : Outport  Port=2  VectorParamsAs1DForOutWhenUnconnected=off
  wires:
  Vdc/1 -> Saturation/1
  Saturation/1 -> Divide/2, Gain2/1
  Gain/1 -> Divide/1
  Sum1/1 -> Saturation1/1  "Duty"
  Sum/1 -> Gain3/1, Product1/1, Bus Creator/2  "M_act"
  Bus Creator/1 -> Mon/1
  Saturation1/1 -> Duty/1, Bus Creator/1  "Duty"
  Constant/1 -> Sum1/2
  Gain3/1 -> Sum1/1
  VabcSp/1 -> Bus Creator/3, Gain/1  "VabcRef"
  Divide/1 -> Square/1, Min/1, Max/1, Sum/1  "M"
  Min/1 -> Add/2
  Max/1 -> Add/1
  Add/1 -> Gain1/1
  Gain1/1 -> Product/2
  Product/1 -> Sum/2
  Relay/1 -> Product/1
  Square/1 -> Discrete Transfer Fcn1/1
  Discrete Transfer Fcn1/1 -> Sqrt/1
  Sqrt/1 -> Relay/1
  Gain2/1 -> Product1/2
  Product1/1 -> Bus Creator/4  "VabcAct"

== system GCI_Ctrl_PLL_C2000/C2000_SW/CtrlLoop/Modulation/SPWM ==
  note: Data Collection
  Vdc : Inport
  VabcSp : Inport  Port=2  OutDataTypeStr=single
  Enable : EnablePort  StatesWhenEnabling=reset
  Bus Creator : BusCreator  Inputs=3
  Constant : Constant  Value=50  OutDataTypeStr=single
  Divide : Product  Inputs=*/
  Divide1 : Product  Inputs=*/
  Gain2 : Gain  Gain=0.5  ParamDataTypeStr=single
  Gain3 : Gain  Gain=50  ParamDataTypeStr=single  OutDataTypeStr=single
  Saturation : Saturate  UpperLimit=50  LowerLimit=-50  OutDataTypeStr=single
  Saturation2 : Saturate  UpperLimit=single(1000)  LowerLimit=single(1)
  Sqrt : Sqrt
  Square : Math  Operator=square
  Subsystem : Subsystem
  Sum of Elements : Sum  Inputs=+
  Sum1 : Sum  Inputs=|++  OutDataTypeStr=single
  Duty : Outport  OutDataTypeStr=single  VectorParamsAs1DForOutWhenUnconnected=off
  Mon : Outport  Port=2  OutDataTypeStr=single  VectorParamsAs1DForOutWhenUnconnected=off
  wires:
  Divide/1 -> Gain3/1  "M_act"
  Constant/1 -> Sum1/2
  Gain3/1 -> Saturation/1
  Sum1/1 -> Bus Creator/1, Duty/1  "Duty"
  Bus Creator/1 -> Mon/1  "ModMon"
  Vdc/1 -> Saturation2/1
  Saturation2/1 -> Gain2/1
  VabcSp/1 -> Bus Creator/3, Divide/1, Subsystem/1(abc)  "VabcRef"
  Saturation/1 -> Sum1/1  "Duty"
  Square/1 -> Sum of Elements/1
  Sum of Elements/1 -> Sqrt/1
  Sqrt/1 -> Divide1/1
  Gain2/1 -> Divide1/2, Divide/2
  Divide1/1 -> Bus Creator/2  "M_act"
  Subsystem/1(al_be_0) -> Square/1

== system GCI_Ctrl_PLL_C2000/C2000_SW/CtrlLoop/Modulation/SVM ==
  note: Data Collection
  Vdc : Inport
  VabcSp : Inport  Port=2
  Enable : EnablePort  StatesWhenEnabling=reset
  Add : Sum
  Bus Creator : BusCreator  Inputs=3
  Constant : Constant  Value=50  OutDataTypeStr=single
  Divide : Product  Inputs=*/
  Gain1 : Gain  Gain=0.5  ParamDataTypeStr=single
  Gain2 : Gain  Gain=0.5  ParamDataTypeStr=single
  Gain3 : Gain  Gain=50  ParamDataTypeStr=single  OutDataTypeStr=single
  Max : MinMax  Function=max
  Min : MinMax
  Saturation : Saturate  UpperLimit=single(1000)  LowerLimit=single(1)
  Saturation1 : Saturate  UpperLimit=100  LowerLimit=0  OutDataTypeStr=single
  Sum : Sum  Inputs=|+-
  Sum1 : Sum  Inputs=|++  OutDataTypeStr=single
  Duty : Outport  VectorParamsAs1DForOutWhenUnconnected=off
  Mon : Outport  Port=2  VectorParamsAs1DForOutWhenUnconnected=off
  wires:
  Gain1/1 -> Sum/2
  Add/1 -> Gain1/1
  Max/1 -> Add/1
  Min/1 -> Add/2
  Divide/1 -> Sum/1, Max/1, Min/1  "M*"
  VabcSp/1 -> Divide/1, Bus Creator/3  "VabcRef"
  Gain3/1 -> Sum1/1
  Constant/1 -> Sum1/2
  Saturation1/1 -> Bus Creator/1, Duty/1  "Duty"
  Bus Creator/1 -> Mon/1
  Sum/1 -> Bus Creator/2, Gain3/1  "M_act"
  Sum1/1 -> Saturation1/1  "Duty"
  Saturation/1 -> Gain2/1
  Vdc/1 -> Saturation/1
  Gain2/1 -> Divide/2

== system GCI_Ctrl_PLL_C2000/C2000_SW/CtrlLoop/Observer/LPF ==
  VabcGrid : Inport
  Discrete Transfer Fcn2 : DiscreteTransferFcn  Numerator=Var.Filt.Sec.num  Denominator=Var.Filt.Sec.den
  Saturation : Saturate  UpperLimit=5  LowerLimit=-5
  Subtract : Sum  Inputs=+-
  VabcGridAdj : Outport  VectorParamsAs1DForOutWhenUnconnected=off
  wires:
  Discrete Transfer Fcn2/1 -> Saturation/1
  VabcGrid/1 -> Subtract/1, Discrete Transfer Fcn2/1
  Subtract/1 -> VabcGridAdj/1
  Saturation/1 -> Subtract/2

== system GCI_Ctrl_PLL_C2000/C2000_SW/CtrlLoop/Observer/LPF1 ==
  VabcGrid : Inport
  Discrete Transfer Fcn2 : DiscreteTransferFcn  Numerator=Var.Filt.Sec.num  Denominator=Var.Filt.Sec.den
  Saturation : Saturate  UpperLimit=5  LowerLimit=-5
  Subtract : Sum  Inputs=+-
  VabcGridAdj : Outport  VectorParamsAs1DForOutWhenUnconnected=off
  wires:
  Saturation/1 -> Subtract/2
  Subtract/1 -> VabcGridAdj/1
  VabcGrid/1 -> Discrete Transfer Fcn2/1, Subtract/1
  Discrete Transfer Fcn2/1 -> Saturation/1

== system GCI_Ctrl_PLL_C2000/C2000_SW/CtrlLoop/PLL_Vref/SRF_PLL ==
  Vdqz : Inport  OutDataTypeStr=single
  Abs1 : Abs  SaturateOnIntegerOverflow=off
  Constant : Constant  Value=0  OutDataTypeStr=single
  Discrete PID Controller : slpidlib/PID Controller  Controller=PI  Form=Parallel  TimeDomain=Discrete-time  UseExternalTs=off  SampleTime=-1  IntegratorMethod=Forward Euler  FilterMethod=Forward Euler  ControllerParametersSource=external  P=1  I=1  UseKiTs=off  D=0  UseExternalDerivativeSource=off  N=100  UseFilter=on  TunerSelectOption=Transfer Function Based (PID Tuner App)  InitialConditionSource=internal  InitialConditionForIntegrator=0  InitialConditionForFilter=0  DifferentiatorICPrevScaledInput=0  ExternalReset=none  TrackingMode=off  Kt=1  LimitOutput=on  SatLimitsSource=internal  UpperSaturationLimit=Var.Pll_MaxDeltaFreq  LowerSaturationLimit=-Var.Pll_MaxDeltaFreq  LinearizeAsGain=on  AntiWindupMode=clamping  Kb=1  LimitIntegrator=off  UpperIntegratorSaturationLimit=inf  LowerIntegratorSaturationLimit=-inf  POutMin=[]  POutMax=[]  IOutMin=[]  IOutMax=[]  DOutMin=[]  DOutMax=[]  NOutMin=[]  NOutMax=[]  SumOutMin=[]  SumOutMax=[]  SaturationOutMin=[]  SaturationOutMax=[]  PParamMin=[]  PParamMax=[]  IParamMin=[]  IParamMax=[]  DParamMin=[]  DParamMax=[]  NParamMin=[]  NParamMax=[]  KbParamMin=[]  KbParamMax=[]  KtParamMin=[]  KtParamMax=[]  KbOutMin=[]  KbOutMax=[]  KtOutMin=[]  KtOutMax=[]  IntegratorOutMin=[]  IntegratorOutMax=[]  FilterOutMin=[]  FilterOutMax=[]  SumI1OutMin=[]  SumI1OutMax=[]  SumI2OutMin=[]  SumI2OutMax=[]  SumI3OutMin=[]  SumI3OutMax=[]  SumI4OutMin=[]  SumI4OutMax=[]  SumDOutMin=[]  SumDOutMax=[]  DifferentiatorOutMin=[]  DifferentiatorOutMax=[]  FilterDiffOutCoefMin=[]  FilterDiffOutCoefMax=[]  ReciprocalOutMin=[]  ReciprocalOutMax=[]  SumDenOutMin=[]  SumDenOutMax=[]  SumNumOutMin=[]  SumNumOutMax=[]  DivideOutMin=[]  DivideOutMax=[]  UdiffTsProdOutMin=[]  UdiffTsProdOutMax=[]  NTsProdOutMin=[]  NTsProdOutMax=[]  UintegralTsProdOutMin=[]  UintegralTsProdOutMax=[]  UngainTsProdOutMin=[]  UngainTsProdOutMax=[]  ClampingZeroOutDataTypeStr=Inherit: Inherit via back propagation  ClampingZeroOutMin=[]  ClampingZeroOutMax=[]  FilterDenConstantOutDataTypeStr=Inherit: Inherit via back propagation  FilterDenConstantOutMin=[]  FilterDenConstantOutMax=[]  PCopyOutDataTypeStr=Inherit: Inherit via back propagation  PCopyOutMin=[]  PCopyOutMax=[]  NCopyOutDataTypeStr=Inherit: Inherit via back propagation  NCopyOutMin=[]  NCopyOutMax=[]  IntegratorContinuousStateAttributes=''  IntegratorStateMustResolveToSignalObject=off  IntegratorRTWStateStorageClass=Auto  FilterContinuousStateAttributes=''  FilterStateMustResolveToSignalObject=off  FilterRTWStateStorageClass=Auto  ParallelPVariant=ExternalParameters  IdealPVariant=Disabled  IVariant=ExternalParameters  DVariant=Disabled  IntegratorVariant=Discrete  SatVariant=Enabled  AWVariant=DiscClampingParallel  PCopyVariant=Disabled  TRVariant=Disabled  FdbkBlocksVariant=Forward  IdealPFdbkVariant=Disabled  SatFdbkVariant=Disabled  DerivativeFilterVariant=Disabled  NVariant=Disabled  NCopyVariant=Disabled_SignalSpec  FilterICVariant=Disabled  IntegratorICVariant=InternalICs  ExternalResetVariant=Disabled  TRSumVariant=Passthrough  SumFdbkVariant=Disabled  SumVariant=Sum_PI  TsampFilterVariant=InternalTs  TsampNgainVariant=Passthrough  TsampIntegralVariant=Disabled_SignalSpec  ExternalSaturationOutDataTypeStr=Inherit: Same as second input  DerivativeSourceVariant=Disabled
  Divide : Product  Inputs=*/
  Gain : Gain  Gain=1/Var.PWM_Freq  ParamDataTypeStr=single
  GridFreq : Constant  Value=single(2*pi*Var.Grid_Frq)  OutDataTypeStr=single
  Ki : Constant  Value=Var.PllKi  OutDataTypeStr=single
  Kp : Constant  Value=Var.PllKp  OutDataTypeStr=single
  LPF : Subsystem  mask{Ts=1/(Var.PWM_Freq), w=single(30), K=single(1), y_0=single(2*pi*Var.Grid_Frq)}
      mask prompts: Ts "Sample Time (s)"; w "CutOff Freq (-3db) (rad/s)"; K "Gain"; y_0 "Initial output"
  LPF1 : Subsystem  mask{Ts=1/(Var.PWM_Freq), w=single(2*pi*10), K=single(1), y_0=single(1)}
      mask prompts: Ts "Sample Time (s)"; w "CutOff Freq (-3db) (rad/s)"; K "Gain"; y_0 "Initial output"
  LPF2 : Subsystem  mask{Ts=1/(Var.PWM_Freq), w=single(2*pi*50), K=single(1), y_0=single(1)}
      mask prompts: Ts "Sample Time (s)"; w "CutOff Freq (-3db) (rad/s)"; K "Gain"; y_0 "Initial output"
  Math Function : Math  Operator=magnitude^2  SignedPower=on
  Relay : Relay  OnSwitchValue=single(0.1)  OffSwitchValue=single(0.05)  OnOutputValue=0  OffOutputValue=1  OutDataTypeStr=boolean
  Saturation : Saturate  UpperLimit=1000  LowerLimit=1
  Selector : Selector  InputPortWidth=3  IndexOptions=Index vector (dialog)  Indices=[2]  OutputSizes=1
  Sqrt : Sqrt
  Sum : Sum  Inputs=|++  OutDataTypeStr=single
  Sum of Elements : Sum  Inputs=+
  Sum1 : Sum  Inputs=++|
  Sum2 : Sum  Inputs=++|  OutDataTypeStr=single
  WrapZeroToTwoPi : Subsystem
  WrapedDiscIntegrator : Subsystem
  wtNext : Outport  OutDataTypeStr=single  VectorParamsAs1DForOutWhenUnconnected=off
  wtNow : Outport  Port=2  OutDataTypeStr=single  VectorParamsAs1DForOutWhenUnconnected=off
  w : Outport  Port=3  OutDataTypeStr=single  VectorParamsAs1DForOutWhenUnconnected=off
  wFilt : Outport  Port=4  OutDataTypeStr=single  VectorParamsAs1DForOutWhenUnconnected=off
  Snch : Outport  Port=5  VectorParamsAs1DForOutWhenUnconnected=off
  wires:
  Ki/1 -> Discrete PID Controller/3
  Discrete PID Controller/1 -> Sum2/2  "PI_Out"
  Sum2/1 -> LPF/1(u), w/1, WrapedDiscIntegrator/1(w)  "w"
  GridFreq/1 -> Sum2/1
  Constant/1 -> Sum/1
  Kp/1 -> Discrete PID Controller/2
  Sum/1 -> Discrete PID Controller/1  "VgQ_PuErr"
  WrapZeroToTwoPi/1(wtWraped) -> wtNext/1  "wtNext"
  LPF/1(y) -> Gain/1, wFilt/1
  Gain/1 -> Sum1/1  "w_Filt_30rad_s_Ts"
  Sum1/1 -> WrapZeroToTwoPi/1(Ang)  "wt_next"
  WrapedDiscIntegrator/1(wt_now) -> wtNow/1, Sum1/2  "wtNow"
  Divide/1 -> Abs1/1, Sum/2  "VgQ_Pu"
  Vdqz/1 -> Math Function/1, Selector/1
  Math Function/1 -> Sum of Elements/1
  Sum of Elements/1 -> Sqrt/1
  Selector/1 -> Divide/1  "VgQ"
  Abs1/1 -> LPF1/1(u)  "VgQ_PuAbs"
  Relay/1 -> Snch/1  "VgQSynch"
  LPF1/1(y) -> Relay/1
  Saturation/1 -> Divide/2
  Sqrt/1 -> LPF2/1(u)
  LPF2/1(y) -> Saturation/1

== system GCI_Ctrl_PLL_C2000/C2000_SW/CtrlLoop/PLL_Vref/Subsystem ==
  Vabc : Inport
  Iabc : Inport  Port=2
  wtNow : Inport  Port=3
  LPF2 : Subsystem  Commented=on  mask{Ts=1/(Var.PWM_Freq), w=single(1000), K=single(1), y_0=0}
      mask prompts: Ts "Sample Time (s)"; w "CutOff Freq (-3db) (rad/s)"; K "Gain"; y_0 "Initial output"
  Mux : Mux  Inputs=2
  PowerCalculation : Subsystem
  Selector{3,5..7} (4 alike) : Selector  InputPortWidth=3  IndexOptions=Index vector (dialog)  Indices=[1 2]  OutputSizes=1
  abc_dqz : Subsystem  VariantControl=Var.Pll.SOGISel == 2
  dd_dqz1 : Subsystem  VariantControl=Var.Pll.SOGISel == 2
  dd_dqz2 : Subsystem  VariantControl=Var.Pll.SOGISel == 2
  PQ : Outport  VectorParamsAs1DForOutWhenUnconnected=off
  Idqz : Outport  Port=2  VectorParamsAs1DForOutWhenUnconnected=off
  wires:
  dd_dqz1/2(dqzN) -> Selector5/1
  PowerCalculation/2(Q0) -> Mux/2  "Q0"
  Selector3/1 -> PowerCalculation/1(VdqP)  "VdqP"
  PowerCalculation/1(P0) -> Mux/1  "P0"
  dd_dqz1/1(dqzP) -> Selector3/1
  Selector7/1 -> PowerCalculation/4(IdqzN)  "IdqN"
  Selector6/1 -> PowerCalculation/3(IdqzP)  "IdqP"
  dd_dqz2/1(dqzP) -> Selector6/1
  Selector5/1 -> PowerCalculation/2(VdqN)  "VdqN"
  dd_dqz2/2(dqzN) -> Selector7/1
  Iabc/1 -> abc_dqz/1(abc), dd_dqz2/1(abc)
  Vabc/1 -> dd_dqz1/1(abc)
  abc_dqz/1(dqz) -> Idqz/1
  wtNow/1 -> abc_dqz/2(wtNow), dd_dqz1/2(wtNow), dd_dqz2/2(wtNow)
  Mux/1 -> PQ/1

== system GCI_Ctrl_PLL_C2000/C2000_SW/CtrlLoop/PLL_Vref/abc2dqzFilt ==
  abc : Inport
  Ang : Inport  Port=2
  w : Inport  Port=3
  Single_SOGI : Subsystem  VariantControl="Sim.SOGISel == \"1P SOGI\""
  dd_dqz : Subsystem  VariantControl="Sim.SOGISel == \"DDSRF\""
  dd_dqz_SOGI : Subsystem  VariantControl="Sim.SOGISel == \"DDSRF SOGI\""
  dqz : Subsystem  VariantControl="Sim.SOGISel == \"SRF\""
  dqz_1P_SOGI_Disc : Subsystem  VariantControl="Sim.SOGISel == \"1P SOGI Disc\""
  dqz_DSOGI : Subsystem  VariantControl="Sim.SOGISel == \"DSOGI\""
  dqz_SOGI : Subsystem  VariantControl="Sim.SOGISel == \"SOGI\""
  dqz_SOGI_ConstW : Subsystem  VariantControl="Sim.SOGISel == \"SOGI Const W\""
  dqz_SOGI_Disc : Subsystem  VariantControl="Sim.SOGISel == \"3P SOGI Disc\""
  Dqz : Outport  VectorParamsAs1DForOutWhenUnconnected=off
  dqz_Pll : Outport  Port=2  VectorParamsAs1DForOutWhenUnconnected=off
